simulink model "SimscapeVCOmodule"  (R2019b)
settings: Solver=VariableStepAuto  StartTime=0.0  StopTime=0.00000005  RelTol=1e-3
model workspace (MAT data in the model file):
  PnFrequencyOffset_42 = [30000 100000 1000000 3000000 10000000]
libraries: fl_lib x3, nesl_utility x2, ee_lib x1
settings Model: Creator=connerhannon  LastModifiedBy=connerhannon

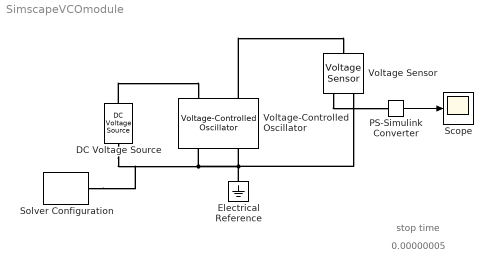
== system SimscapeVCOmodule ==
  note: stop time
  note: 0.00000005
  DC Voltage Source : fl_lib/Electrical/Electrical Sources/DC Voltage Source  v0=0 V
  Electrical Reference : fl_lib/Electrical/Electrical Elements/Electrical Reference
  PS-Simulink Converter : nesl_utility/PS-Simulink Converter  PhysicalDomain=network_engine_domain  SubClassName=ps_output  LeftPortType=input  RightPortType=output  PseudoPeriodic=off  Frequencies=[]  Unit=inherit  AffineConversion=off
  Scope : Scope
  Solver Configuration : nesl_utility/Solver Configuration  PhysicalDomain=network_engine_domain  SubClassName=solver  LeftPortType=input  RightPortType=generic  Tones=[]  Harmonics=[]  SimulateNoise=off  Profile=off  UseLocalSampling=off  EnableSwitchedLinearOptims=on  FrequencyDomain=off  UseCCode=off  RelTol=0.001  AbsTol=1e-06  MinStep=1e-09  ToWorkspace=off  RevertToSquareIcSolve=off  NumHomotopyIterations=100  PhasorMode=off  PhasorModeNumHarmonics=1  DoDC=off  ResidualTolerance=1e-09  UseLocalSolver=off  LocalSolverChoice=NE_BACKWARD_EULER_ADVANCER  LocalSolverSampleTime=0.001  DoFixedCost=off  MaxNonlinIter=3  MaxModeIter=2  LinearAlgebra=auto  EquationFormulation=NE_TIME_EF  DelaysMemoryBudget=1024  AutomaticFiltering=on  FilteringTimeConstant=0.001  PartitionStorageMethod=AS_NEEDED  PartitionMemoryBudget=1024  PartitionMethod=ROBUST
  Voltage Sensor : fl_lib/Electrical/Electrical Sensors/Voltage Sensor
  Voltage-Controlled Oscillator : ee_lib/Integrated Circuits/Voltage-Controlled Oscillator  tabulated=1  f_nom=31.33 MHz  v_nom=0.5 V  df_dv=1 Hz/V  v_min=0 V  v_max=1 V  v_vec=|  f_vec=[0, 0.98, 1.82, 2.47, 3.05, 3.56, 4.04, 4.44, 4.8, 5.17, 5.46, 5.75, 6, 6.26, 6.48, 6.66, 6.84, 6.99, 7.13, 7.28, 7.39, 7.49, 7.6, 7.68, 7.75, 7.82] MHz  v_out=1 V  r_in=inf Ohm  r_out=0 Ohm  model_dynamics=0  time_constant=1e-3 s  f_ini=1000 Hz
      | [0, 0.2, 0.4, 0.6, 0.8, 1, 1.2, 1.4, 1.6, 1.8, 2, 2.2, 2.4, 2.6, 2.8, 3, 3.2, 3.4, 3.6, 3.8, 4, 4.2, 4.4, 4.6, 4.8, 5]
      |  V
      settings: SourceProductName=Simscape Electrical  SourceProductBaseCode=PS  InternalSimscapePortConfiguration="{\"Bottom\":[],\"Left\":[{\"id\":\"p1\",\"label\":\"1+\",\"type\":\"foundation.electrical.electrical\"},{\"id\":\"p2\",\"label\":\"2+\",\"type\":\"foundation.electrical.electrical\"}],\"Right\":[{\"id\":\"n1\",\"label\":\"1-\",\"type\":\"foundation.electrical.electrical\"},{\"id\":\"n2\",\"label\":\"2-\",\"type\":\"foundation.electrical.electrical\"}],\"Top\":[]}"
  wires:
  PS-Simulink Converter/1 -> Scope/1
  connections:
  Electrical Reference/LConn1 -- Solver Configuration/RConn1 -- DC Voltage Source/RConn1 -- Voltage-Controlled Oscillator/RConn1 -- Voltage Sensor/RConn2 -- Voltage-Controlled Oscillator/RConn2
  DC Voltage Source/LConn1 -- Voltage-Controlled Oscillator/LConn1
  Voltage-Controlled Oscillator/LConn2 -- Voltage Sensor/LConn1
  Voltage Sensor/RConn1 -- PS-Simulink Converter/LConn1
